simulink model "wt_multi"  (R2022b)
settings: Solver=FixedStepDiscrete  StartTime=0.0  StopTime=10.0  RelTol=1e-3
PreLoadFcn:
  | addpath('/nfs/ug/homes-1/z/zha13325/ece1718/a2_k/a2_hw/hdlimport/wt_multi');
libraries: simulink x2808, hdlsllib x1459
(part 10 of 22)

== system wt_multi/wt_multi/ca04/fa18 ==
  in1 : Inport  OutDataTypeStr=fixdt(0, 1, 0)  SampleTime=-1
  in2 : Inport  Port=2  OutDataTypeStr=fixdt(0, 1, 0)  SampleTime=-1
  Cin : Inport  Port=3  OutDataTypeStr=fixdt(0, 1, 0)  SampleTime=-1
  Bit_AND : simulink/Logic and Bit Operations/Bitwise Operator  logicop=AND  UseBitMask=off  NumInputPorts=2  BitMask=double(0)  BitMaskRealWorld=Real World Value
  Bit_AND_1 : simulink/Logic and Bit Operations/Bitwise Operator  logicop=AND  UseBitMask=off  NumInputPorts=2  BitMask=double(0)  BitMaskRealWorld=Real World Value
  Bit_OR : simulink/Logic and Bit Operations/Bitwise Operator  logicop=OR  UseBitMask=off  NumInputPorts=2  BitMask=double(0)  BitMaskRealWorld=Real World Value
  Bit_XOR : simulink/Logic and Bit Operations/Bitwise Operator  logicop=XOR  UseBitMask=off  NumInputPorts=2  BitMask=double(0)  BitMaskRealWorld=Real World Value
  Bit_XOR_1 : simulink/Logic and Bit Operations/Bitwise Operator  logicop=XOR  UseBitMask=off  NumInputPorts=2  BitMask=double(0)  BitMaskRealWorld=Real World Value
  Bit_XOR_2 : simulink/Logic and Bit Operations/Bitwise Operator  logicop=XOR  UseBitMask=off  NumInputPorts=2  BitMask=double(0)  BitMaskRealWorld=Real World Value
  S : Outport  OutDataTypeStr=fixdt(0, 1, 0)  SampleTime=-1
  C : Outport  Port=2  OutDataTypeStr=fixdt(0, 1, 0)  SampleTime=-1
  wires:
  in2/1 -> Bit_XOR_2/2, Bit_AND/2, Bit_XOR_1/2
  Cin/1 -> Bit_AND_1/1, Bit_XOR/2
  Bit_AND_1/1 -> Bit_OR/2
  in1/1 -> Bit_XOR_2/1, Bit_AND/1, Bit_XOR_1/1
  Bit_OR/1 -> C/1
  Bit_XOR_2/1 -> Bit_AND_1/2
  Bit_XOR/1 -> S/1
  Bit_AND/1 -> Bit_OR/1
  Bit_XOR_1/1 -> Bit_XOR/1

== system wt_multi/wt_multi/ca04/fa19 ==
  in1 : Inport  OutDataTypeStr=fixdt(0, 1, 0)  SampleTime=-1
  in2 : Inport  Port=2  OutDataTypeStr=fixdt(0, 1, 0)  SampleTime=-1
  Cin : Inport  Port=3  OutDataTypeStr=fixdt(0, 1, 0)  SampleTime=-1
  Bit_AND : simulink/Logic and Bit Operations/Bitwise Operator  logicop=AND  UseBitMask=off  NumInputPorts=2  BitMask=double(0)  BitMaskRealWorld=Real World Value
  Bit_AND_1 : simulink/Logic and Bit Operations/Bitwise Operator  logicop=AND  UseBitMask=off  NumInputPorts=2  BitMask=double(0)  BitMaskRealWorld=Real World Value
  Bit_OR : simulink/Logic and Bit Operations/Bitwise Operator  logicop=OR  UseBitMask=off  NumInputPorts=2  BitMask=double(0)  BitMaskRealWorld=Real World Value
  Bit_XOR : simulink/Logic and Bit Operations/Bitwise Operator  logicop=XOR  UseBitMask=off  NumInputPorts=2  BitMask=double(0)  BitMaskRealWorld=Real World Value
  Bit_XOR_1 : simulink/Logic and Bit Operations/Bitwise Operator  logicop=XOR  UseBitMask=off  NumInputPorts=2  BitMask=double(0)  BitMaskRealWorld=Real World Value
  Bit_XOR_2 : simulink/Logic and Bit Operations/Bitwise Operator  logicop=XOR  UseBitMask=off  NumInputPorts=2  BitMask=double(0)  BitMaskRealWorld=Real World Value
  S : Outport  OutDataTypeStr=fixdt(0, 1, 0)  SampleTime=-1
  C : Outport  Port=2  OutDataTypeStr=fixdt(0, 1, 0)  SampleTime=-1
  wires:
  in1/1 -> Bit_XOR_2/1, Bit_AND/1, Bit_XOR_1/1
  in2/1 -> Bit_XOR_2/2, Bit_AND/2, Bit_XOR_1/2
  Cin/1 -> Bit_AND_1/1, Bit_XOR/2
  Bit_AND_1/1 -> Bit_OR/2
  Bit_OR/1 -> C/1
  Bit_XOR_2/1 -> Bit_AND_1/2
  Bit_XOR/1 -> S/1
  Bit_AND/1 -> Bit_OR/1
  Bit_XOR_1/1 -> Bit_XOR/1

== system wt_multi/wt_multi/ca04/fa2 ==
  in1 : Inport  OutDataTypeStr=fixdt(0, 1, 0)  SampleTime=-1
  in2 : Inport  Port=2  OutDataTypeStr=fixdt(0, 1, 0)  SampleTime=-1
  Cin : Inport  Port=3  OutDataTypeStr=fixdt(0, 1, 0)  SampleTime=-1
  Bit_AND : simulink/Logic and Bit Operations/Bitwise Operator  logicop=AND  UseBitMask=off  NumInputPorts=2  BitMask=double(0)  BitMaskRealWorld=Real World Value
  Bit_AND_1 : simulink/Logic and Bit Operations/Bitwise Operator  logicop=AND  UseBitMask=off  NumInputPorts=2  BitMask=double(0)  BitMaskRealWorld=Real World Value
  Bit_OR : simulink/Logic and Bit Operations/Bitwise Operator  logicop=OR  UseBitMask=off  NumInputPorts=2  BitMask=double(0)  BitMaskRealWorld=Real World Value
  Bit_XOR : simulink/Logic and Bit Operations/Bitwise Operator  logicop=XOR  UseBitMask=off  NumInputPorts=2  BitMask=double(0)  BitMaskRealWorld=Real World Value
  Bit_XOR_1 : simulink/Logic and Bit Operations/Bitwise Operator  logicop=XOR  UseBitMask=off  NumInputPorts=2  BitMask=double(0)  BitMaskRealWorld=Real World Value
  Bit_XOR_2 : simulink/Logic and Bit Operations/Bitwise Operator  logicop=XOR  UseBitMask=off  NumInputPorts=2  BitMask=double(0)  BitMaskRealWorld=Real World Value
  S : Outport  OutDataTypeStr=fixdt(0, 1, 0)  SampleTime=-1
  C : Outport  Port=2  OutDataTypeStr=fixdt(0, 1, 0)  SampleTime=-1
  wires:
  in1/1 -> Bit_XOR_2/1, Bit_AND/1, Bit_XOR_1/1
  in2/1 -> Bit_XOR_2/2, Bit_AND/2, Bit_XOR_1/2
  Cin/1 -> Bit_AND_1/1, Bit_XOR/2
  Bit_AND_1/1 -> Bit_OR/2
  Bit_OR/1 -> C/1
  Bit_XOR_2/1 -> Bit_AND_1/2
  Bit_AND/1 -> Bit_OR/1
  Bit_XOR_1/1 -> Bit_XOR/1
  Bit_XOR/1 -> S/1

== system wt_multi/wt_multi/ca04/fa20 ==
  in1 : Inport  OutDataTypeStr=fixdt(0, 1, 0)  SampleTime=-1
  in2 : Inport  Port=2  OutDataTypeStr=fixdt(0, 1, 0)  SampleTime=-1
  Cin : Inport  Port=3  OutDataTypeStr=fixdt(0, 1, 0)  SampleTime=-1
  Bit_AND : simulink/Logic and Bit Operations/Bitwise Operator  logicop=AND  UseBitMask=off  NumInputPorts=2  BitMask=double(0)  BitMaskRealWorld=Real World Value
  Bit_AND_1 : simulink/Logic and Bit Operations/Bitwise Operator  logicop=AND  UseBitMask=off  NumInputPorts=2  BitMask=double(0)  BitMaskRealWorld=Real World Value
  Bit_OR : simulink/Logic and Bit Operations/Bitwise Operator  logicop=OR  UseBitMask=off  NumInputPorts=2  BitMask=double(0)  BitMaskRealWorld=Real World Value
  Bit_XOR : simulink/Logic and Bit Operations/Bitwise Operator  logicop=XOR  UseBitMask=off  NumInputPorts=2  BitMask=double(0)  BitMaskRealWorld=Real World Value
  Bit_XOR_1 : simulink/Logic and Bit Operations/Bitwise Operator  logicop=XOR  UseBitMask=off  NumInputPorts=2  BitMask=double(0)  BitMaskRealWorld=Real World Value
  Bit_XOR_2 : simulink/Logic and Bit Operations/Bitwise Operator  logicop=XOR  UseBitMask=off  NumInputPorts=2  BitMask=double(0)  BitMaskRealWorld=Real World Value
  S : Outport  OutDataTypeStr=fixdt(0, 1, 0)  SampleTime=-1
  C : Outport  Port=2  OutDataTypeStr=fixdt(0, 1, 0)  SampleTime=-1
  wires:
  in2/1 -> Bit_XOR_2/2, Bit_AND/2, Bit_XOR_1/2
  Bit_AND_1/1 -> Bit_OR/2
  Bit_OR/1 -> C/1
  Bit_XOR_1/1 -> Bit_XOR/1
  Bit_XOR_2/1 -> Bit_AND_1/2
  in1/1 -> Bit_XOR_2/1, Bit_AND/1, Bit_XOR_1/1
  Bit_AND/1 -> Bit_OR/1
  Cin/1 -> Bit_AND_1/1, Bit_XOR/2
  Bit_XOR/1 -> S/1

== system wt_multi/wt_multi/ca04/fa21 ==
  in1 : Inport  OutDataTypeStr=fixdt(0, 1, 0)  SampleTime=-1
  in2 : Inport  Port=2  OutDataTypeStr=fixdt(0, 1, 0)  SampleTime=-1
  Cin : Inport  Port=3  OutDataTypeStr=fixdt(0, 1, 0)  SampleTime=-1
  Bit_AND : simulink/Logic and Bit Operations/Bitwise Operator  logicop=AND  UseBitMask=off  NumInputPorts=2  BitMask=double(0)  BitMaskRealWorld=Real World Value
  Bit_AND_1 : simulink/Logic and Bit Operations/Bitwise Operator  logicop=AND  UseBitMask=off  NumInputPorts=2  BitMask=double(0)  BitMaskRealWorld=Real World Value
  Bit_OR : simulink/Logic and Bit Operations/Bitwise Operator  logicop=OR  UseBitMask=off  NumInputPorts=2  BitMask=double(0)  BitMaskRealWorld=Real World Value
  Bit_XOR : simulink/Logic and Bit Operations/Bitwise Operator  logicop=XOR  UseBitMask=off  NumInputPorts=2  BitMask=double(0)  BitMaskRealWorld=Real World Value
  Bit_XOR_1 : simulink/Logic and Bit Operations/Bitwise Operator  logicop=XOR  UseBitMask=off  NumInputPorts=2  BitMask=double(0)  BitMaskRealWorld=Real World Value
  Bit_XOR_2 : simulink/Logic and Bit Operations/Bitwise Operator  logicop=XOR  UseBitMask=off  NumInputPorts=2  BitMask=double(0)  BitMaskRealWorld=Real World Value
  S : Outport  OutDataTypeStr=fixdt(0, 1, 0)  SampleTime=-1
  C : Outport  Port=2  OutDataTypeStr=fixdt(0, 1, 0)  SampleTime=-1
  wires:
  in1/1 -> Bit_XOR_2/1, Bit_AND/1, Bit_XOR_1/1
  in2/1 -> Bit_XOR_2/2, Bit_AND/2, Bit_XOR_1/2
  Cin/1 -> Bit_AND_1/1, Bit_XOR/2
  Bit_AND_1/1 -> Bit_OR/2
  Bit_OR/1 -> C/1
  Bit_XOR_2/1 -> Bit_AND_1/2
  Bit_AND/1 -> Bit_OR/1
  Bit_XOR/1 -> S/1
  Bit_XOR_1/1 -> Bit_XOR/1

== system wt_multi/wt_multi/ca04/fa22 ==
  in1 : Inport  OutDataTypeStr=fixdt(0, 1, 0)  SampleTime=-1
  in2 : Inport  Port=2  OutDataTypeStr=fixdt(0, 1, 0)  SampleTime=-1
  Cin : Inport  Port=3  OutDataTypeStr=fixdt(0, 1, 0)  SampleTime=-1
  Bit_AND : simulink/Logic and Bit Operations/Bitwise Operator  logicop=AND  UseBitMask=off  NumInputPorts=2  BitMask=double(0)  BitMaskRealWorld=Real World Value
  Bit_AND_1 : simulink/Logic and Bit Operations/Bitwise Operator  logicop=AND  UseBitMask=off  NumInputPorts=2  BitMask=double(0)  BitMaskRealWorld=Real World Value
  Bit_OR : simulink/Logic and Bit Operations/Bitwise Operator  logicop=OR  UseBitMask=off  NumInputPorts=2  BitMask=double(0)  BitMaskRealWorld=Real World Value
  Bit_XOR : simulink/Logic and Bit Operations/Bitwise Operator  logicop=XOR  UseBitMask=off  NumInputPorts=2  BitMask=double(0)  BitMaskRealWorld=Real World Value
  Bit_XOR_1 : simulink/Logic and Bit Operations/Bitwise Operator  logicop=XOR  UseBitMask=off  NumInputPorts=2  BitMask=double(0)  BitMaskRealWorld=Real World Value
  Bit_XOR_2 : simulink/Logic and Bit Operations/Bitwise Operator  logicop=XOR  UseBitMask=off  NumInputPorts=2  BitMask=double(0)  BitMaskRealWorld=Real World Value
  S : Outport  OutDataTypeStr=fixdt(0, 1, 0)  SampleTime=-1
  C : Outport  Port=2  OutDataTypeStr=fixdt(0, 1, 0)  SampleTime=-1
  wires:
  in1/1 -> Bit_XOR_2/1, Bit_AND/1, Bit_XOR_1/1
  in2/1 -> Bit_XOR_2/2, Bit_AND/2, Bit_XOR_1/2
  Bit_AND_1/1 -> Bit_OR/2
  Bit_OR/1 -> C/1
  Cin/1 -> Bit_AND_1/1, Bit_XOR/2
  Bit_AND/1 -> Bit_OR/1
  Bit_XOR_2/1 -> Bit_AND_1/2
  Bit_XOR/1 -> S/1
  Bit_XOR_1/1 -> Bit_XOR/1

== system wt_multi/wt_multi/ca04/fa23 ==
  in1 : Inport  OutDataTypeStr=fixdt(0, 1, 0)  SampleTime=-1
  in2 : Inport  Port=2  OutDataTypeStr=fixdt(0, 1, 0)  SampleTime=-1
  Cin : Inport  Port=3  OutDataTypeStr=fixdt(0, 1, 0)  SampleTime=-1
  Bit_AND : simulink/Logic and Bit Operations/Bitwise Operator  logicop=AND  UseBitMask=off  NumInputPorts=2  BitMask=double(0)  BitMaskRealWorld=Real World Value
  Bit_AND_1 : simulink/Logic and Bit Operations/Bitwise Operator  logicop=AND  UseBitMask=off  NumInputPorts=2  BitMask=double(0)  BitMaskRealWorld=Real World Value
  Bit_OR : simulink/Logic and Bit Operations/Bitwise Operator  logicop=OR  UseBitMask=off  NumInputPorts=2  BitMask=double(0)  BitMaskRealWorld=Real World Value
  Bit_XOR : simulink/Logic and Bit Operations/Bitwise Operator  logicop=XOR  UseBitMask=off  NumInputPorts=2  BitMask=double(0)  BitMaskRealWorld=Real World Value
  Bit_XOR_1 : simulink/Logic and Bit Operations/Bitwise Operator  logicop=XOR  UseBitMask=off  NumInputPorts=2  BitMask=double(0)  BitMaskRealWorld=Real World Value
  Bit_XOR_2 : simulink/Logic and Bit Operations/Bitwise Operator  logicop=XOR  UseBitMask=off  NumInputPorts=2  BitMask=double(0)  BitMaskRealWorld=Real World Value
  S : Outport  OutDataTypeStr=fixdt(0, 1, 0)  SampleTime=-1
  C : Outport  Port=2  OutDataTypeStr=fixdt(0, 1, 0)  SampleTime=-1
  wires:
  in1/1 -> Bit_XOR_2/1, Bit_AND/1, Bit_XOR_1/1
  in2/1 -> Bit_XOR_2/2, Bit_AND/2, Bit_XOR_1/2
  Bit_AND_1/1 -> Bit_OR/2
  Bit_OR/1 -> C/1
  Bit_XOR_2/1 -> Bit_AND_1/2
  Bit_XOR_1/1 -> Bit_XOR/1
  Cin/1 -> Bit_AND_1/1, Bit_XOR/2
  Bit_AND/1 -> Bit_OR/1
  Bit_XOR/1 -> S/1

== system wt_multi/wt_multi/ca04/fa24 ==
  in1 : Inport  OutDataTypeStr=fixdt(0, 1, 0)  SampleTime=-1
  in2 : Inport  Port=2  OutDataTypeStr=fixdt(0, 1, 0)  SampleTime=-1
  Cin : Inport  Port=3  OutDataTypeStr=fixdt(0, 1, 0)  SampleTime=-1
  Bit_AND : simulink/Logic and Bit Operations/Bitwise Operator  logicop=AND  UseBitMask=off  NumInputPorts=2  BitMask=double(0)  BitMaskRealWorld=Real World Value
  Bit_AND_1 : simulink/Logic and Bit Operations/Bitwise Operator  logicop=AND  UseBitMask=off  NumInputPorts=2  BitMask=double(0)  BitMaskRealWorld=Real World Value
  Bit_OR : simulink/Logic and Bit Operations/Bitwise Operator  logicop=OR  UseBitMask=off  NumInputPorts=2  BitMask=double(0)  BitMaskRealWorld=Real World Value
  Bit_XOR : simulink/Logic and Bit Operations/Bitwise Operator  logicop=XOR  UseBitMask=off  NumInputPorts=2  BitMask=double(0)  BitMaskRealWorld=Real World Value
  Bit_XOR_1 : simulink/Logic and Bit Operations/Bitwise Operator  logicop=XOR  UseBitMask=off  NumInputPorts=2  BitMask=double(0)  BitMaskRealWorld=Real World Value
  Bit_XOR_2 : simulink/Logic and Bit Operations/Bitwise Operator  logicop=XOR  UseBitMask=off  NumInputPorts=2  BitMask=double(0)  BitMaskRealWorld=Real World Value
  S : Outport  OutDataTypeStr=fixdt(0, 1, 0)  SampleTime=-1
  C : Outport  Port=2  OutDataTypeStr=fixdt(0, 1, 0)  SampleTime=-1
  wires:
  in1/1 -> Bit_XOR_2/1, Bit_AND/1, Bit_XOR_1/1
  Cin/1 -> Bit_AND_1/1, Bit_XOR/2
  Bit_AND_1/1 -> Bit_OR/2
  Bit_XOR_1/1 -> Bit_XOR/1
  in2/1 -> Bit_XOR_2/2, Bit_AND/2, Bit_XOR_1/2
  Bit_OR/1 -> C/1
  Bit_XOR/1 -> S/1
  Bit_XOR_2/1 -> Bit_AND_1/2
  Bit_AND/1 -> Bit_OR/1

== system wt_multi/wt_multi/ca04/fa25 ==
  in1 : Inport  OutDataTypeStr=fixdt(0, 1, 0)  SampleTime=-1
  in2 : Inport  Port=2  OutDataTypeStr=fixdt(0, 1, 0)  SampleTime=-1
  Cin : Inport  Port=3  OutDataTypeStr=fixdt(0, 1, 0)  SampleTime=-1
  Bit_AND : simulink/Logic and Bit Operations/Bitwise Operator  logicop=AND  UseBitMask=off  NumInputPorts=2  BitMask=double(0)  BitMaskRealWorld=Real World Value
  Bit_AND_1 : simulink/Logic and Bit Operations/Bitwise Operator  logicop=AND  UseBitMask=off  NumInputPorts=2  BitMask=double(0)  BitMaskRealWorld=Real World Value
  Bit_OR : simulink/Logic and Bit Operations/Bitwise Operator  logicop=OR  UseBitMask=off  NumInputPorts=2  BitMask=double(0)  BitMaskRealWorld=Real World Value
  Bit_XOR : simulink/Logic and Bit Operations/Bitwise Operator  logicop=XOR  UseBitMask=off  NumInputPorts=2  BitMask=double(0)  BitMaskRealWorld=Real World Value
  Bit_XOR_1 : simulink/Logic and Bit Operations/Bitwise Operator  logicop=XOR  UseBitMask=off  NumInputPorts=2  BitMask=double(0)  BitMaskRealWorld=Real World Value
  Bit_XOR_2 : simulink/Logic and Bit Operations/Bitwise Operator  logicop=XOR  UseBitMask=off  NumInputPorts=2  BitMask=double(0)  BitMaskRealWorld=Real World Value
  S : Outport  OutDataTypeStr=fixdt(0, 1, 0)  SampleTime=-1
  C : Outport  Port=2  OutDataTypeStr=fixdt(0, 1, 0)  SampleTime=-1
  wires:
  in1/1 -> Bit_XOR_2/1, Bit_AND/1, Bit_XOR_1/1
  in2/1 -> Bit_XOR_2/2, Bit_AND/2, Bit_XOR_1/2
  Cin/1 -> Bit_AND_1/1, Bit_XOR/2
  Bit_AND_1/1 -> Bit_OR/2
  Bit_AND/1 -> Bit_OR/1
  Bit_OR/1 -> C/1
  Bit_XOR_1/1 -> Bit_XOR/1
  Bit_XOR_2/1 -> Bit_AND_1/2
  Bit_XOR/1 -> S/1

== system wt_multi/wt_multi/ca04/fa26 ==
  in1 : Inport  OutDataTypeStr=fixdt(0, 1, 0)  SampleTime=-1
  in2 : Inport  Port=2  OutDataTypeStr=fixdt(0, 1, 0)  SampleTime=-1
  Cin : Inport  Port=3  OutDataTypeStr=fixdt(0, 1, 0)  SampleTime=-1
  Bit_AND : simulink/Logic and Bit Operations/Bitwise Operator  logicop=AND  UseBitMask=off  NumInputPorts=2  BitMask=double(0)  BitMaskRealWorld=Real World Value
  Bit_AND_1 : simulink/Logic and Bit Operations/Bitwise Operator  logicop=AND  UseBitMask=off  NumInputPorts=2  BitMask=double(0)  BitMaskRealWorld=Real World Value
  Bit_OR : simulink/Logic and Bit Operations/Bitwise Operator  logicop=OR  UseBitMask=off  NumInputPorts=2  BitMask=double(0)  BitMaskRealWorld=Real World Value
  Bit_XOR : simulink/Logic and Bit Operations/Bitwise Operator  logicop=XOR  UseBitMask=off  NumInputPorts=2  BitMask=double(0)  BitMaskRealWorld=Real World Value
  Bit_XOR_1 : simulink/Logic and Bit Operations/Bitwise Operator  logicop=XOR  UseBitMask=off  NumInputPorts=2  BitMask=double(0)  BitMaskRealWorld=Real World Value
  Bit_XOR_2 : simulink/Logic and Bit Operations/Bitwise Operator  logicop=XOR  UseBitMask=off  NumInputPorts=2  BitMask=double(0)  BitMaskRealWorld=Real World Value
  S : Outport  OutDataTypeStr=fixdt(0, 1, 0)  SampleTime=-1
  C : Outport  Port=2  OutDataTypeStr=fixdt(0, 1, 0)  SampleTime=-1
  wires:
  in1/1 -> Bit_XOR_2/1, Bit_AND/1, Bit_XOR_1/1
  in2/1 -> Bit_XOR_2/2, Bit_AND/2, Bit_XOR_1/2
  Cin/1 -> Bit_AND_1/1, Bit_XOR/2
  Bit_OR/1 -> C/1
  Bit_AND/1 -> Bit_OR/1
  Bit_XOR/1 -> S/1
  Bit_AND_1/1 -> Bit_OR/2
  Bit_XOR_2/1 -> Bit_AND_1/2
  Bit_XOR_1/1 -> Bit_XOR/1

== system wt_multi/wt_multi/ca04/fa27 ==
  in1 : Inport  OutDataTypeStr=fixdt(0, 1, 0)  SampleTime=-1
  in2 : Inport  Port=2  OutDataTypeStr=fixdt(0, 1, 0)  SampleTime=-1
  Cin : Inport  Port=3  OutDataTypeStr=fixdt(0, 1, 0)  SampleTime=-1
  Bit_AND : simulink/Logic and Bit Operations/Bitwise Operator  logicop=AND  UseBitMask=off  NumInputPorts=2  BitMask=double(0)  BitMaskRealWorld=Real World Value
  Bit_AND_1 : simulink/Logic and Bit Operations/Bitwise Operator  logicop=AND  UseBitMask=off  NumInputPorts=2  BitMask=double(0)  BitMaskRealWorld=Real World Value
  Bit_OR : simulink/Logic and Bit Operations/Bitwise Operator  logicop=OR  UseBitMask=off  NumInputPorts=2  BitMask=double(0)  BitMaskRealWorld=Real World Value
  Bit_XOR : simulink/Logic and Bit Operations/Bitwise Operator  logicop=XOR  UseBitMask=off  NumInputPorts=2  BitMask=double(0)  BitMaskRealWorld=Real World Value
  Bit_XOR_1 : simulink/Logic and Bit Operations/Bitwise Operator  logicop=XOR  UseBitMask=off  NumInputPorts=2  BitMask=double(0)  BitMaskRealWorld=Real World Value
  Bit_XOR_2 : simulink/Logic and Bit Operations/Bitwise Operator  logicop=XOR  UseBitMask=off  NumInputPorts=2  BitMask=double(0)  BitMaskRealWorld=Real World Value
  S : Outport  OutDataTypeStr=fixdt(0, 1, 0)  SampleTime=-1
  C : Outport  Port=2  OutDataTypeStr=fixdt(0, 1, 0)  SampleTime=-1
  wires:
  in1/1 -> Bit_XOR_2/1, Bit_AND/1, Bit_XOR_1/1
  in2/1 -> Bit_XOR_2/2, Bit_AND/2, Bit_XOR_1/2
  Cin/1 -> Bit_AND_1/1, Bit_XOR/2
  Bit_AND_1/1 -> Bit_OR/2
  Bit_XOR_2/1 -> Bit_AND_1/2
  Bit_OR/1 -> C/1
  Bit_XOR_1/1 -> Bit_XOR/1
  Bit_AND/1 -> Bit_OR/1
  Bit_XOR/1 -> S/1

== system wt_multi/wt_multi/ca04/fa28 ==
  in1 : Inport  OutDataTypeStr=fixdt(0, 1, 0)  SampleTime=-1
  in2 : Inport  Port=2  OutDataTypeStr=fixdt(0, 1, 0)  SampleTime=-1
  Cin : Inport  Port=3  OutDataTypeStr=fixdt(0, 1, 0)  SampleTime=-1
  Bit_AND : simulink/Logic and Bit Operations/Bitwise Operator  logicop=AND  UseBitMask=off  NumInputPorts=2  BitMask=double(0)  BitMaskRealWorld=Real World Value
  Bit_AND_1 : simulink/Logic and Bit Operations/Bitwise Operator  logicop=AND  UseBitMask=off  NumInputPorts=2  BitMask=double(0)  BitMaskRealWorld=Real World Value
  Bit_OR : simulink/Logic and Bit Operations/Bitwise Operator  logicop=OR  UseBitMask=off  NumInputPorts=2  BitMask=double(0)  BitMaskRealWorld=Real World Value
  Bit_XOR : simulink/Logic and Bit Operations/Bitwise Operator  logicop=XOR  UseBitMask=off  NumInputPorts=2  BitMask=double(0)  BitMaskRealWorld=Real World Value
  Bit_XOR_1 : simulink/Logic and Bit Operations/Bitwise Operator  logicop=XOR  UseBitMask=off  NumInputPorts=2  BitMask=double(0)  BitMaskRealWorld=Real World Value
  Bit_XOR_2 : simulink/Logic and Bit Operations/Bitwise Operator  logicop=XOR  UseBitMask=off  NumInputPorts=2  BitMask=double(0)  BitMaskRealWorld=Real World Value
  S : Outport  OutDataTypeStr=fixdt(0, 1, 0)  SampleTime=-1
  C : Outport  Port=2  OutDataTypeStr=fixdt(0, 1, 0)  SampleTime=-1
  wires:
  Cin/1 -> Bit_AND_1/1, Bit_XOR/2
  Bit_AND/1 -> Bit_OR/1
  Bit_OR/1 -> C/1
  in1/1 -> Bit_XOR_2/1, Bit_AND/1, Bit_XOR_1/1
  Bit_AND_1/1 -> Bit_OR/2
  Bit_XOR_2/1 -> Bit_AND_1/2
  Bit_XOR/1 -> S/1
  in2/1 -> Bit_XOR_2/2, Bit_AND/2, Bit_XOR_1/2
  Bit_XOR_1/1 -> Bit_XOR/1

== system wt_multi/wt_multi/ca04/fa29 ==
  in1 : Inport  OutDataTypeStr=fixdt(0, 1, 0)  SampleTime=-1
  in2 : Inport  Port=2  OutDataTypeStr=fixdt(0, 1, 0)  SampleTime=-1
  Cin : Inport  Port=3  OutDataTypeStr=fixdt(0, 1, 0)  SampleTime=-1
  Bit_AND : simulink/Logic and Bit Operations/Bitwise Operator  logicop=AND  UseBitMask=off  NumInputPorts=2  BitMask=double(0)  BitMaskRealWorld=Real World Value
  Bit_AND_1 : simulink/Logic and Bit Operations/Bitwise Operator  logicop=AND  UseBitMask=off  NumInputPorts=2  BitMask=double(0)  BitMaskRealWorld=Real World Value
  Bit_OR : simulink/Logic and Bit Operations/Bitwise Operator  logicop=OR  UseBitMask=off  NumInputPorts=2  BitMask=double(0)  BitMaskRealWorld=Real World Value
  Bit_XOR : simulink/Logic and Bit Operations/Bitwise Operator  logicop=XOR  UseBitMask=off  NumInputPorts=2  BitMask=double(0)  BitMaskRealWorld=Real World Value
  Bit_XOR_1 : simulink/Logic and Bit Operations/Bitwise Operator  logicop=XOR  UseBitMask=off  NumInputPorts=2  BitMask=double(0)  BitMaskRealWorld=Real World Value
  Bit_XOR_2 : simulink/Logic and Bit Operations/Bitwise Operator  logicop=XOR  UseBitMask=off  NumInputPorts=2  BitMask=double(0)  BitMaskRealWorld=Real World Value
  S : Outport  OutDataTypeStr=fixdt(0, 1, 0)  SampleTime=-1
  C : Outport  Port=2  OutDataTypeStr=fixdt(0, 1, 0)  SampleTime=-1
  wires:
  in2/1 -> Bit_XOR_2/2, Bit_AND/2, Bit_XOR_1/2
  Cin/1 -> Bit_AND_1/1, Bit_XOR/2
  Bit_AND/1 -> Bit_OR/1
  Bit_AND_1/1 -> Bit_OR/2
  Bit_OR/1 -> C/1
  Bit_XOR/1 -> S/1
  in1/1 -> Bit_XOR_2/1, Bit_AND/1, Bit_XOR_1/1
  Bit_XOR_2/1 -> Bit_AND_1/2
  Bit_XOR_1/1 -> Bit_XOR/1

== system wt_multi/wt_multi/ca04/fa3 ==
  in1 : Inport  OutDataTypeStr=fixdt(0, 1, 0)  SampleTime=-1
  in2 : Inport  Port=2  OutDataTypeStr=fixdt(0, 1, 0)  SampleTime=-1
  Cin : Inport  Port=3  OutDataTypeStr=fixdt(0, 1, 0)  SampleTime=-1
  Bit_AND : simulink/Logic and Bit Operations/Bitwise Operator  logicop=AND  UseBitMask=off  NumInputPorts=2  BitMask=double(0)  BitMaskRealWorld=Real World Value
  Bit_AND_1 : simulink/Logic and Bit Operations/Bitwise Operator  logicop=AND  UseBitMask=off  NumInputPorts=2  BitMask=double(0)  BitMaskRealWorld=Real World Value
  Bit_OR : simulink/Logic and Bit Operations/Bitwise Operator  logicop=OR  UseBitMask=off  NumInputPorts=2  BitMask=double(0)  BitMaskRealWorld=Real World Value
  Bit_XOR : simulink/Logic and Bit Operations/Bitwise Operator  logicop=XOR  UseBitMask=off  NumInputPorts=2  BitMask=double(0)  BitMaskRealWorld=Real World Value
  Bit_XOR_1 : simulink/Logic and Bit Operations/Bitwise Operator  logicop=XOR  UseBitMask=off  NumInputPorts=2  BitMask=double(0)  BitMaskRealWorld=Real World Value
  Bit_XOR_2 : simulink/Logic and Bit Operations/Bitwise Operator  logicop=XOR  UseBitMask=off  NumInputPorts=2  BitMask=double(0)  BitMaskRealWorld=Real World Value
  S : Outport  OutDataTypeStr=fixdt(0, 1, 0)  SampleTime=-1
  C : Outport  Port=2  OutDataTypeStr=fixdt(0, 1, 0)  SampleTime=-1
  wires:
  in1/1 -> Bit_XOR_2/1, Bit_AND/1, Bit_XOR_1/1
  Cin/1 -> Bit_AND_1/1, Bit_XOR/2
  Bit_AND_1/1 -> Bit_OR/2
  Bit_XOR_2/1 -> Bit_AND_1/2
  Bit_OR/1 -> C/1
  in2/1 -> Bit_XOR_2/2, Bit_AND/2, Bit_XOR_1/2
  Bit_XOR/1 -> S/1
  Bit_XOR_1/1 -> Bit_XOR/1
  Bit_AND/1 -> Bit_OR/1

== system wt_multi/wt_multi/ca04/fa30 ==
  in1 : Inport  OutDataTypeStr=fixdt(0, 1, 0)  SampleTime=-1
  in2 : Inport  Port=2  OutDataTypeStr=fixdt(0, 1, 0)  SampleTime=-1
  Cin : Inport  Port=3  OutDataTypeStr=fixdt(0, 1, 0)  SampleTime=-1
  Bit_AND : simulink/Logic and Bit Operations/Bitwise Operator  logicop=AND  UseBitMask=off  NumInputPorts=2  BitMask=double(0)  BitMaskRealWorld=Real World Value
  Bit_AND_1 : simulink/Logic and Bit Operations/Bitwise Operator  logicop=AND  UseBitMask=off  NumInputPorts=2  BitMask=double(0)  BitMaskRealWorld=Real World Value
  Bit_OR : simulink/Logic and Bit Operations/Bitwise Operator  logicop=OR  UseBitMask=off  NumInputPorts=2  BitMask=double(0)  BitMaskRealWorld=Real World Value
  Bit_XOR : simulink/Logic and Bit Operations/Bitwise Operator  logicop=XOR  UseBitMask=off  NumInputPorts=2  BitMask=double(0)  BitMaskRealWorld=Real World Value
  Bit_XOR_1 : simulink/Logic and Bit Operations/Bitwise Operator  logicop=XOR  UseBitMask=off  NumInputPorts=2  BitMask=double(0)  BitMaskRealWorld=Real World Value
  Bit_XOR_2 : simulink/Logic and Bit Operations/Bitwise Operator  logicop=XOR  UseBitMask=off  NumInputPorts=2  BitMask=double(0)  BitMaskRealWorld=Real World Value
  S : Outport  OutDataTypeStr=fixdt(0, 1, 0)  SampleTime=-1
  C : Outport  Port=2  OutDataTypeStr=fixdt(0, 1, 0)  SampleTime=-1
  wires:
  in1/1 -> Bit_XOR_2/1, Bit_AND/1, Bit_XOR_1/1
  in2/1 -> Bit_XOR_2/2, Bit_AND/2, Bit_XOR_1/2
  Cin/1 -> Bit_AND_1/1, Bit_XOR/2
  Bit_AND_1/1 -> Bit_OR/2
  Bit_OR/1 -> C/1
  Bit_XOR_1/1 -> Bit_XOR/1
  Bit_XOR_2/1 -> Bit_AND_1/2
  Bit_AND/1 -> Bit_OR/1
  Bit_XOR/1 -> S/1

== system wt_multi/wt_multi/ca04/fa4 ==
  in1 : Inport  OutDataTypeStr=fixdt(0, 1, 0)  SampleTime=-1
  in2 : Inport  Port=2  OutDataTypeStr=fixdt(0, 1, 0)  SampleTime=-1
  Cin : Inport  Port=3  OutDataTypeStr=fixdt(0, 1, 0)  SampleTime=-1
  Bit_AND : simulink/Logic and Bit Operations/Bitwise Operator  logicop=AND  UseBitMask=off  NumInputPorts=2  BitMask=double(0)  BitMaskRealWorld=Real World Value
  Bit_AND_1 : simulink/Logic and Bit Operations/Bitwise Operator  logicop=AND  UseBitMask=off  NumInputPorts=2  BitMask=double(0)  BitMaskRealWorld=Real World Value
  Bit_OR : simulink/Logic and Bit Operations/Bitwise Operator  logicop=OR  UseBitMask=off  NumInputPorts=2  BitMask=double(0)  BitMaskRealWorld=Real World Value
  Bit_XOR : simulink/Logic and Bit Operations/Bitwise Operator  logicop=XOR  UseBitMask=off  NumInputPorts=2  BitMask=double(0)  BitMaskRealWorld=Real World Value
  Bit_XOR_1 : simulink/Logic and Bit Operations/Bitwise Operator  logicop=XOR  UseBitMask=off  NumInputPorts=2  BitMask=double(0)  BitMaskRealWorld=Real World Value
  Bit_XOR_2 : simulink/Logic and Bit Operations/Bitwise Operator  logicop=XOR  UseBitMask=off  NumInputPorts=2  BitMask=double(0)  BitMaskRealWorld=Real World Value
  S : Outport  OutDataTypeStr=fixdt(0, 1, 0)  SampleTime=-1
  C : Outport  Port=2  OutDataTypeStr=fixdt(0, 1, 0)  SampleTime=-1
  wires:
  Cin/1 -> Bit_AND_1/1, Bit_XOR/2
  Bit_AND_1/1 -> Bit_OR/2
  Bit_OR/1 -> C/1
  Bit_XOR_2/1 -> Bit_AND_1/2
  Bit_AND/1 -> Bit_OR/1
  in1/1 -> Bit_XOR_2/1, Bit_AND/1, Bit_XOR_1/1
  in2/1 -> Bit_XOR_2/2, Bit_AND/2, Bit_XOR_1/2
  Bit_XOR/1 -> S/1
  Bit_XOR_1/1 -> Bit_XOR/1

== system wt_multi/wt_multi/ca04/fa5 ==
  in1 : Inport  OutDataTypeStr=fixdt(0, 1, 0)  SampleTime=-1
  in2 : Inport  Port=2  OutDataTypeStr=fixdt(0, 1, 0)  SampleTime=-1
  Cin : Inport  Port=3  OutDataTypeStr=fixdt(0, 1, 0)  SampleTime=-1
  Bit_AND : simulink/Logic and Bit Operations/Bitwise Operator  logicop=AND  UseBitMask=off  NumInputPorts=2  BitMask=double(0)  BitMaskRealWorld=Real World Value
  Bit_AND_1 : simulink/Logic and Bit Operations/Bitwise Operator  logicop=AND  UseBitMask=off  NumInputPorts=2  BitMask=double(0)  BitMaskRealWorld=Real World Value
  Bit_OR : simulink/Logic and Bit Operations/Bitwise Operator  logicop=OR  UseBitMask=off  NumInputPorts=2  BitMask=double(0)  BitMaskRealWorld=Real World Value
  Bit_XOR : simulink/Logic and Bit Operations/Bitwise Operator  logicop=XOR  UseBitMask=off  NumInputPorts=2  BitMask=double(0)  BitMaskRealWorld=Real World Value
  Bit_XOR_1 : simulink/Logic and Bit Operations/Bitwise Operator  logicop=XOR  UseBitMask=off  NumInputPorts=2  BitMask=double(0)  BitMaskRealWorld=Real World Value
  Bit_XOR_2 : simulink/Logic and Bit Operations/Bitwise Operator  logicop=XOR  UseBitMask=off  NumInputPorts=2  BitMask=double(0)  BitMaskRealWorld=Real World Value
  S : Outport  OutDataTypeStr=fixdt(0, 1, 0)  SampleTime=-1
  C : Outport  Port=2  OutDataTypeStr=fixdt(0, 1, 0)  SampleTime=-1
  wires:
  in2/1 -> Bit_XOR_2/2, Bit_AND/2, Bit_XOR_1/2
  Cin/1 -> Bit_AND_1/1, Bit_XOR/2
  Bit_AND_1/1 -> Bit_OR/2
  Bit_OR/1 -> C/1
  Bit_XOR_2/1 -> Bit_AND_1/2
  in1/1 -> Bit_XOR_2/1, Bit_AND/1, Bit_XOR_1/1
  Bit_AND/1 -> Bit_OR/1
  Bit_XOR_1/1 -> Bit_XOR/1
  Bit_XOR/1 -> S/1

== system wt_multi/wt_multi/ca04/fa6 ==
  in1 : Inport  OutDataTypeStr=fixdt(0, 1, 0)  SampleTime=-1
  in2 : Inport  Port=2  OutDataTypeStr=fixdt(0, 1, 0)  SampleTime=-1
  Cin : Inport  Port=3  OutDataTypeStr=fixdt(0, 1, 0)  SampleTime=-1
  Bit_AND : simulink/Logic and Bit Operations/Bitwise Operator  logicop=AND  UseBitMask=off  NumInputPorts=2  BitMask=double(0)  BitMaskRealWorld=Real World Value
  Bit_AND_1 : simulink/Logic and Bit Operations/Bitwise Operator  logicop=AND  UseBitMask=off  NumInputPorts=2  BitMask=double(0)  BitMaskRealWorld=Real World Value
  Bit_OR : simulink/Logic and Bit Operations/Bitwise Operator  logicop=OR  UseBitMask=off  NumInputPorts=2  BitMask=double(0)  BitMaskRealWorld=Real World Value
  Bit_XOR : simulink/Logic and Bit Operations/Bitwise Operator  logicop=XOR  UseBitMask=off  NumInputPorts=2  BitMask=double(0)  BitMaskRealWorld=Real World Value
  Bit_XOR_1 : simulink/Logic and Bit Operations/Bitwise Operator  logicop=XOR  UseBitMask=off  NumInputPorts=2  BitMask=double(0)  BitMaskRealWorld=Real World Value
  Bit_XOR_2 : simulink/Logic and Bit Operations/Bitwise Operator  logicop=XOR  UseBitMask=off  NumInputPorts=2  BitMask=double(0)  BitMaskRealWorld=Real World Value
  S : Outport  OutDataTypeStr=fixdt(0, 1, 0)  SampleTime=-1
  C : Outport  Port=2  OutDataTypeStr=fixdt(0, 1, 0)  SampleTime=-1
  wires:
  in1/1 -> Bit_XOR_2/1, Bit_AND/1, Bit_XOR_1/1
  Bit_AND_1/1 -> Bit_OR/2
  in2/1 -> Bit_XOR_2/2, Bit_AND/2, Bit_XOR_1/2
  Cin/1 -> Bit_AND_1/1, Bit_XOR/2
  Bit_OR/1 -> C/1
  Bit_XOR_2/1 -> Bit_AND_1/2
  Bit_AND/1 -> Bit_OR/1
  Bit_XOR/1 -> S/1
  Bit_XOR_1/1 -> Bit_XOR/1

== system wt_multi/wt_multi/ca04/fa7 ==
  in1 : Inport  OutDataTypeStr=fixdt(0, 1, 0)  SampleTime=-1
  in2 : Inport  Port=2  OutDataTypeStr=fixdt(0, 1, 0)  SampleTime=-1
  Cin : Inport  Port=3  OutDataTypeStr=fixdt(0, 1, 0)  SampleTime=-1
  Bit_AND : simulink/Logic and Bit Operations/Bitwise Operator  logicop=AND  UseBitMask=off  NumInputPorts=2  BitMask=double(0)  BitMaskRealWorld=Real World Value
  Bit_AND_1 : simulink/Logic and Bit Operations/Bitwise Operator  logicop=AND  UseBitMask=off  NumInputPorts=2  BitMask=double(0)  BitMaskRealWorld=Real World Value
  Bit_OR : simulink/Logic and Bit Operations/Bitwise Operator  logicop=OR  UseBitMask=off  NumInputPorts=2  BitMask=double(0)  BitMaskRealWorld=Real World Value
  Bit_XOR : simulink/Logic and Bit Operations/Bitwise Operator  logicop=XOR  UseBitMask=off  NumInputPorts=2  BitMask=double(0)  BitMaskRealWorld=Real World Value
  Bit_XOR_1 : simulink/Logic and Bit Operations/Bitwise Operator  logicop=XOR  UseBitMask=off  NumInputPorts=2  BitMask=double(0)  BitMaskRealWorld=Real World Value
  Bit_XOR_2 : simulink/Logic and Bit Operations/Bitwise Operator  logicop=XOR  UseBitMask=off  NumInputPorts=2  BitMask=double(0)  BitMaskRealWorld=Real World Value
  S : Outport  OutDataTypeStr=fixdt(0, 1, 0)  SampleTime=-1
  C : Outport  Port=2  OutDataTypeStr=fixdt(0, 1, 0)  SampleTime=-1
  wires:
  in1/1 -> Bit_XOR_2/1, Bit_AND/1, Bit_XOR_1/1
  in2/1 -> Bit_XOR_2/2, Bit_AND/2, Bit_XOR_1/2
  Cin/1 -> Bit_AND_1/1, Bit_XOR/2
  Bit_AND_1/1 -> Bit_OR/2
  Bit_OR/1 -> C/1
  Bit_XOR_2/1 -> Bit_AND_1/2
  Bit_XOR_1/1 -> Bit_XOR/1
  Bit_AND/1 -> Bit_OR/1
  Bit_XOR/1 -> S/1

== system wt_multi/wt_multi/ca04/fa8 ==
  in1 : Inport  OutDataTypeStr=fixdt(0, 1, 0)  SampleTime=-1
  in2 : Inport  Port=2  OutDataTypeStr=fixdt(0, 1, 0)  SampleTime=-1
  Cin : Inport  Port=3  OutDataTypeStr=fixdt(0, 1, 0)  SampleTime=-1
  Bit_AND : simulink/Logic and Bit Operations/Bitwise Operator  logicop=AND  UseBitMask=off  NumInputPorts=2  BitMask=double(0)  BitMaskRealWorld=Real World Value
  Bit_AND_1 : simulink/Logic and Bit Operations/Bitwise Operator  logicop=AND  UseBitMask=off  NumInputPorts=2  BitMask=double(0)  BitMaskRealWorld=Real World Value
  Bit_OR : simulink/Logic and Bit Operations/Bitwise Operator  logicop=OR  UseBitMask=off  NumInputPorts=2  BitMask=double(0)  BitMaskRealWorld=Real World Value
  Bit_XOR : simulink/Logic and Bit Operations/Bitwise Operator  logicop=XOR  UseBitMask=off  NumInputPorts=2  BitMask=double(0)  BitMaskRealWorld=Real World Value
  Bit_XOR_1 : simulink/Logic and Bit Operations/Bitwise Operator  logicop=XOR  UseBitMask=off  NumInputPorts=2  BitMask=double(0)  BitMaskRealWorld=Real World Value
  Bit_XOR_2 : simulink/Logic and Bit Operations/Bitwise Operator  logicop=XOR  UseBitMask=off  NumInputPorts=2  BitMask=double(0)  BitMaskRealWorld=Real World Value
  S : Outport  OutDataTypeStr=fixdt(0, 1, 0)  SampleTime=-1
  C : Outport  Port=2  OutDataTypeStr=fixdt(0, 1, 0)  SampleTime=-1
  wires:
  in1/1 -> Bit_XOR_2/1, Bit_AND/1, Bit_XOR_1/1
  Cin/1 -> Bit_AND_1/1, Bit_XOR/2
  Bit_AND_1/1 -> Bit_OR/2
  in2/1 -> Bit_XOR_2/2, Bit_AND/2, Bit_XOR_1/2
  Bit_AND/1 -> Bit_OR/1
  Bit_OR/1 -> C/1
  Bit_XOR_2/1 -> Bit_AND_1/2
  Bit_XOR/1 -> S/1
  Bit_XOR_1/1 -> Bit_XOR/1

== system wt_multi/wt_multi/ca04/fa9 ==
  in1 : Inport  OutDataTypeStr=fixdt(0, 1, 0)  SampleTime=-1
  in2 : Inport  Port=2  OutDataTypeStr=fixdt(0, 1, 0)  SampleTime=-1
  Cin : Inport  Port=3  OutDataTypeStr=fixdt(0, 1, 0)  SampleTime=-1
  Bit_AND : simulink/Logic and Bit Operations/Bitwise Operator  logicop=AND  UseBitMask=off  NumInputPorts=2  BitMask=double(0)  BitMaskRealWorld=Real World Value
  Bit_AND_1 : simulink/Logic and Bit Operations/Bitwise Operator  logicop=AND  UseBitMask=off  NumInputPorts=2  BitMask=double(0)  BitMaskRealWorld=Real World Value
  Bit_OR : simulink/Logic and Bit Operations/Bitwise Operator  logicop=OR  UseBitMask=off  NumInputPorts=2  BitMask=double(0)  BitMaskRealWorld=Real World Value
  Bit_XOR : simulink/Logic and Bit Operations/Bitwise Operator  logicop=XOR  UseBitMask=off  NumInputPorts=2  BitMask=double(0)  BitMaskRealWorld=Real World Value
  Bit_XOR_1 : simulink/Logic and Bit Operations/Bitwise Operator  logicop=XOR  UseBitMask=off  NumInputPorts=2  BitMask=double(0)  BitMaskRealWorld=Real World Value
  Bit_XOR_2 : simulink/Logic and Bit Operations/Bitwise Operator  logicop=XOR  UseBitMask=off  NumInputPorts=2  BitMask=double(0)  BitMaskRealWorld=Real World Value
  S : Outport  OutDataTypeStr=fixdt(0, 1, 0)  SampleTime=-1
  C : Outport  Port=2  OutDataTypeStr=fixdt(0, 1, 0)  SampleTime=-1
  wires:
  in1/1 -> Bit_XOR_2/1, Bit_AND/1, Bit_XOR_1/1
  Cin/1 -> Bit_AND_1/1, Bit_XOR/2
  Bit_AND_1/1 -> Bit_OR/2
  Bit_OR/1 -> C/1
  in2/1 -> Bit_XOR_2/2, Bit_AND/2, Bit_XOR_1/2
  Bit_AND/1 -> Bit_OR/1
  Bit_XOR_2/1 -> Bit_AND_1/2
  Bit_XOR/1 -> S/1
  Bit_XOR_1/1 -> Bit_XOR/1

== system wt_multi/wt_multi/ca05/fa ==
  in1 : Inport  OutDataTypeStr=fixdt(0, 1, 0)  SampleTime=-1
  in2 : Inport  Port=2  OutDataTypeStr=fixdt(0, 1, 0)  SampleTime=-1
  Cin : Inport  Port=3  OutDataTypeStr=fixdt(0, 1, 0)  SampleTime=-1
  Bit_AND : simulink/Logic and Bit Operations/Bitwise Operator  logicop=AND  UseBitMask=off  NumInputPorts=2  BitMask=double(0)  BitMaskRealWorld=Real World Value
  Bit_AND_1 : simulink/Logic and Bit Operations/Bitwise Operator  logicop=AND  UseBitMask=off  NumInputPorts=2  BitMask=double(0)  BitMaskRealWorld=Real World Value
  Bit_OR : simulink/Logic and Bit Operations/Bitwise Operator  logicop=OR  UseBitMask=off  NumInputPorts=2  BitMask=double(0)  BitMaskRealWorld=Real World Value
  Bit_XOR : simulink/Logic and Bit Operations/Bitwise Operator  logicop=XOR  UseBitMask=off  NumInputPorts=2  BitMask=double(0)  BitMaskRealWorld=Real World Value
  Bit_XOR_1 : simulink/Logic and Bit Operations/Bitwise Operator  logicop=XOR  UseBitMask=off  NumInputPorts=2  BitMask=double(0)  BitMaskRealWorld=Real World Value
  Bit_XOR_2 : simulink/Logic and Bit Operations/Bitwise Operator  logicop=XOR  UseBitMask=off  NumInputPorts=2  BitMask=double(0)  BitMaskRealWorld=Real World Value
  S : Outport  OutDataTypeStr=fixdt(0, 1, 0)  SampleTime=-1
  C : Outport  Port=2  OutDataTypeStr=fixdt(0, 1, 0)  SampleTime=-1
  wires:
  in1/1 -> Bit_XOR_2/1, Bit_AND/1, Bit_XOR_1/1
  in2/1 -> Bit_XOR_2/2, Bit_AND/2, Bit_XOR_1/2
  Cin/1 -> Bit_AND_1/1, Bit_XOR/2
  Bit_AND_1/1 -> Bit_OR/2
  Bit_OR/1 -> C/1
  Bit_XOR_2/1 -> Bit_AND_1/2
  Bit_XOR/1 -> S/1
  Bit_AND/1 -> Bit_OR/1
  Bit_XOR_1/1 -> Bit_XOR/1

== system wt_multi/wt_multi/ca05/fa1 ==
  in1 : Inport  OutDataTypeStr=fixdt(0, 1, 0)  SampleTime=-1
  in2 : Inport  Port=2  OutDataTypeStr=fixdt(0, 1, 0)  SampleTime=-1
  Cin : Inport  Port=3  OutDataTypeStr=fixdt(0, 1, 0)  SampleTime=-1
  Bit_AND : simulink/Logic and Bit Operations/Bitwise Operator  logicop=AND  UseBitMask=off  NumInputPorts=2  BitMask=double(0)  BitMaskRealWorld=Real World Value
  Bit_AND_1 : simulink/Logic and Bit Operations/Bitwise Operator  logicop=AND  UseBitMask=off  NumInputPorts=2  BitMask=double(0)  BitMaskRealWorld=Real World Value
  Bit_OR : simulink/Logic and Bit Operations/Bitwise Operator  logicop=OR  UseBitMask=off  NumInputPorts=2  BitMask=double(0)  BitMaskRealWorld=Real World Value
  Bit_XOR : simulink/Logic and Bit Operations/Bitwise Operator  logicop=XOR  UseBitMask=off  NumInputPorts=2  BitMask=double(0)  BitMaskRealWorld=Real World Value
  Bit_XOR_1 : simulink/Logic and Bit Operations/Bitwise Operator  logicop=XOR  UseBitMask=off  NumInputPorts=2  BitMask=double(0)  BitMaskRealWorld=Real World Value
  Bit_XOR_2 : simulink/Logic and Bit Operations/Bitwise Operator  logicop=XOR  UseBitMask=off  NumInputPorts=2  BitMask=double(0)  BitMaskRealWorld=Real World Value
  S : Outport  OutDataTypeStr=fixdt(0, 1, 0)  SampleTime=-1
  C : Outport  Port=2  OutDataTypeStr=fixdt(0, 1, 0)  SampleTime=-1
  wires:
  in1/1 -> Bit_XOR_2/1, Bit_AND/1, Bit_XOR_1/1
  in2/1 -> Bit_XOR_2/2, Bit_AND/2, Bit_XOR_1/2
  Cin/1 -> Bit_AND_1/1, Bit_XOR/2
  Bit_AND_1/1 -> Bit_OR/2
  Bit_OR/1 -> C/1
  Bit_AND/1 -> Bit_OR/1
  Bit_XOR_2/1 -> Bit_AND_1/2
  Bit_XOR/1 -> S/1
  Bit_XOR_1/1 -> Bit_XOR/1

== system wt_multi/wt_multi/ca05/fa10 ==
  in1 : Inport  OutDataTypeStr=fixdt(0, 1, 0)  SampleTime=-1
  in2 : Inport  Port=2  OutDataTypeStr=fixdt(0, 1, 0)  SampleTime=-1
  Cin : Inport  Port=3  OutDataTypeStr=fixdt(0, 1, 0)  SampleTime=-1
  Bit_AND : simulink/Logic and Bit Operations/Bitwise Operator  logicop=AND  UseBitMask=off  NumInputPorts=2  BitMask=double(0)  BitMaskRealWorld=Real World Value
  Bit_AND_1 : simulink/Logic and Bit Operations/Bitwise Operator  logicop=AND  UseBitMask=off  NumInputPorts=2  BitMask=double(0)  BitMaskRealWorld=Real World Value
  Bit_OR : simulink/Logic and Bit Operations/Bitwise Operator  logicop=OR  UseBitMask=off  NumInputPorts=2  BitMask=double(0)  BitMaskRealWorld=Real World Value
  Bit_XOR : simulink/Logic and Bit Operations/Bitwise Operator  logicop=XOR  UseBitMask=off  NumInputPorts=2  BitMask=double(0)  BitMaskRealWorld=Real World Value
  Bit_XOR_1 : simulink/Logic and Bit Operations/Bitwise Operator  logicop=XOR  UseBitMask=off  NumInputPorts=2  BitMask=double(0)  BitMaskRealWorld=Real World Value
  Bit_XOR_2 : simulink/Logic and Bit Operations/Bitwise Operator  logicop=XOR  UseBitMask=off  NumInputPorts=2  BitMask=double(0)  BitMaskRealWorld=Real World Value
  S : Outport  OutDataTypeStr=fixdt(0, 1, 0)  SampleTime=-1
  C : Outport  Port=2  OutDataTypeStr=fixdt(0, 1, 0)  SampleTime=-1
  wires:
  Cin/1 -> Bit_AND_1/1, Bit_XOR/2
  in2/1 -> Bit_XOR_2/2, Bit_AND/2, Bit_XOR_1/2
  Bit_AND_1/1 -> Bit_OR/2
  Bit_AND/1 -> Bit_OR/1
  Bit_XOR_2/1 -> Bit_AND_1/2
  Bit_XOR/1 -> S/1
  in1/1 -> Bit_XOR_2/1, Bit_AND/1, Bit_XOR_1/1
  Bit_OR/1 -> C/1
  Bit_XOR_1/1 -> Bit_XOR/1

== system wt_multi/wt_multi/ca05/fa11 ==
  in1 : Inport  OutDataTypeStr=fixdt(0, 1, 0)  SampleTime=-1
  in2 : Inport  Port=2  OutDataTypeStr=fixdt(0, 1, 0)  SampleTime=-1
  Cin : Inport  Port=3  OutDataTypeStr=fixdt(0, 1, 0)  SampleTime=-1
  Bit_AND : simulink/Logic and Bit Operations/Bitwise Operator  logicop=AND  UseBitMask=off  NumInputPorts=2  BitMask=double(0)  BitMaskRealWorld=Real World Value
  Bit_AND_1 : simulink/Logic and Bit Operations/Bitwise Operator  logicop=AND  UseBitMask=off  NumInputPorts=2  BitMask=double(0)  BitMaskRealWorld=Real World Value
  Bit_OR : simulink/Logic and Bit Operations/Bitwise Operator  logicop=OR  UseBitMask=off  NumInputPorts=2  BitMask=double(0)  BitMaskRealWorld=Real World Value
  Bit_XOR : simulink/Logic and Bit Operations/Bitwise Operator  logicop=XOR  UseBitMask=off  NumInputPorts=2  BitMask=double(0)  BitMaskRealWorld=Real World Value
  Bit_XOR_1 : simulink/Logic and Bit Operations/Bitwise Operator  logicop=XOR  UseBitMask=off  NumInputPorts=2  BitMask=double(0)  BitMaskRealWorld=Real World Value
  Bit_XOR_2 : simulink/Logic and Bit Operations/Bitwise Operator  logicop=XOR  UseBitMask=off  NumInputPorts=2  BitMask=double(0)  BitMaskRealWorld=Real World Value
  S : Outport  OutDataTypeStr=fixdt(0, 1, 0)  SampleTime=-1
  C : Outport  Port=2  OutDataTypeStr=fixdt(0, 1, 0)  SampleTime=-1
  wires:
  in1/1 -> Bit_XOR_2/1, Bit_AND/1, Bit_XOR_1/1
  in2/1 -> Bit_XOR_2/2, Bit_AND/2, Bit_XOR_1/2
  Cin/1 -> Bit_AND_1/1, Bit_XOR/2
  Bit_AND_1/1 -> Bit_OR/2
  Bit_OR/1 -> C/1
  Bit_XOR_2/1 -> Bit_AND_1/2
  Bit_AND/1 -> Bit_OR/1
  Bit_XOR/1 -> S/1
  Bit_XOR_1/1 -> Bit_XOR/1

== system wt_multi/wt_multi/ca05/fa12 ==
  in1 : Inport  OutDataTypeStr=fixdt(0, 1, 0)  SampleTime=-1
  in2 : Inport  Port=2  OutDataTypeStr=fixdt(0, 1, 0)  SampleTime=-1
  Cin : Inport  Port=3  OutDataTypeStr=fixdt(0, 1, 0)  SampleTime=-1
  Bit_AND : simulink/Logic and Bit Operations/Bitwise Operator  logicop=AND  UseBitMask=off  NumInputPorts=2  BitMask=double(0)  BitMaskRealWorld=Real World Value
  Bit_AND_1 : simulink/Logic and Bit Operations/Bitwise Operator  logicop=AND  UseBitMask=off  NumInputPorts=2  BitMask=double(0)  BitMaskRealWorld=Real World Value
  Bit_OR : simulink/Logic and Bit Operations/Bitwise Operator  logicop=OR  UseBitMask=off  NumInputPorts=2  BitMask=double(0)  BitMaskRealWorld=Real World Value
  Bit_XOR : simulink/Logic and Bit Operations/Bitwise Operator  logicop=XOR  UseBitMask=off  NumInputPorts=2  BitMask=double(0)  BitMaskRealWorld=Real World Value
  Bit_XOR_1 : simulink/Logic and Bit Operations/Bitwise Operator  logicop=XOR  UseBitMask=off  NumInputPorts=2  BitMask=double(0)  BitMaskRealWorld=Real World Value
  Bit_XOR_2 : simulink/Logic and Bit Operations/Bitwise Operator  logicop=XOR  UseBitMask=off  NumInputPorts=2  BitMask=double(0)  BitMaskRealWorld=Real World Value
  S : Outport  OutDataTypeStr=fixdt(0, 1, 0)  SampleTime=-1
  C : Outport  Port=2  OutDataTypeStr=fixdt(0, 1, 0)  SampleTime=-1
  wires:
  in2/1 -> Bit_XOR_2/2, Bit_AND/2, Bit_XOR_1/2
  Cin/1 -> Bit_AND_1/1, Bit_XOR/2
  in1/1 -> Bit_XOR_2/1, Bit_AND/1, Bit_XOR_1/1
  Bit_AND_1/1 -> Bit_OR/2
  Bit_XOR/1 -> S/1
  Bit_OR/1 -> C/1
  Bit_XOR_2/1 -> Bit_AND_1/2
  Bit_AND/1 -> Bit_OR/1
  Bit_XOR_1/1 -> Bit_XOR/1

== system wt_multi/wt_multi/ca05/fa13 ==
  in1 : Inport  OutDataTypeStr=fixdt(0, 1, 0)  SampleTime=-1
  in2 : Inport  Port=2  OutDataTypeStr=fixdt(0, 1, 0)  SampleTime=-1
  Cin : Inport  Port=3  OutDataTypeStr=fixdt(0, 1, 0)  SampleTime=-1
  Bit_AND : simulink/Logic and Bit Operations/Bitwise Operator  logicop=AND  UseBitMask=off  NumInputPorts=2  BitMask=double(0)  BitMaskRealWorld=Real World Value
  Bit_AND_1 : simulink/Logic and Bit Operations/Bitwise Operator  logicop=AND  UseBitMask=off  NumInputPorts=2  BitMask=double(0)  BitMaskRealWorld=Real World Value
  Bit_OR : simulink/Logic and Bit Operations/Bitwise Operator  logicop=OR  UseBitMask=off  NumInputPorts=2  BitMask=double(0)  BitMaskRealWorld=Real World Value
  Bit_XOR : simulink/Logic and Bit Operations/Bitwise Operator  logicop=XOR  UseBitMask=off  NumInputPorts=2  BitMask=double(0)  BitMaskRealWorld=Real World Value
  Bit_XOR_1 : simulink/Logic and Bit Operations/Bitwise Operator  logicop=XOR  UseBitMask=off  NumInputPorts=2  BitMask=double(0)  BitMaskRealWorld=Real World Value
  Bit_XOR_2 : simulink/Logic and Bit Operations/Bitwise Operator  logicop=XOR  UseBitMask=off  NumInputPorts=2  BitMask=double(0)  BitMaskRealWorld=Real World Value
  S : Outport  OutDataTypeStr=fixdt(0, 1, 0)  SampleTime=-1
  C : Outport  Port=2  OutDataTypeStr=fixdt(0, 1, 0)  SampleTime=-1
  wires:
  in1/1 -> Bit_XOR_2/1, Bit_AND/1, Bit_XOR_1/1
  in2/1 -> Bit_XOR_2/2, Bit_AND/2, Bit_XOR_1/2
  Cin/1 -> Bit_AND_1/1, Bit_XOR/2
  Bit_AND_1/1 -> Bit_OR/2
  Bit_OR/1 -> C/1
  Bit_XOR_1/1 -> Bit_XOR/1
  Bit_XOR_2/1 -> Bit_AND_1/2
  Bit_AND/1 -> Bit_OR/1
  Bit_XOR/1 -> S/1

== system wt_multi/wt_multi/ca05/fa14 ==
  in1 : Inport  OutDataTypeStr=fixdt(0, 1, 0)  SampleTime=-1
  in2 : Inport  Port=2  OutDataTypeStr=fixdt(0, 1, 0)  SampleTime=-1
  Cin : Inport  Port=3  OutDataTypeStr=fixdt(0, 1, 0)  SampleTime=-1
  Bit_AND : simulink/Logic and Bit Operations/Bitwise Operator  logicop=AND  UseBitMask=off  NumInputPorts=2  BitMask=double(0)  BitMaskRealWorld=Real World Value
  Bit_AND_1 : simulink/Logic and Bit Operations/Bitwise Operator  logicop=AND  UseBitMask=off  NumInputPorts=2  BitMask=double(0)  BitMaskRealWorld=Real World Value
  Bit_OR : simulink/Logic and Bit Operations/Bitwise Operator  logicop=OR  UseBitMask=off  NumInputPorts=2  BitMask=double(0)  BitMaskRealWorld=Real World Value
  Bit_XOR : simulink/Logic and Bit Operations/Bitwise Operator  logicop=XOR  UseBitMask=off  NumInputPorts=2  BitMask=double(0)  BitMaskRealWorld=Real World Value
  Bit_XOR_1 : simulink/Logic and Bit Operations/Bitwise Operator  logicop=XOR  UseBitMask=off  NumInputPorts=2  BitMask=double(0)  BitMaskRealWorld=Real World Value
  Bit_XOR_2 : simulink/Logic and Bit Operations/Bitwise Operator  logicop=XOR  UseBitMask=off  NumInputPorts=2  BitMask=double(0)  BitMaskRealWorld=Real World Value
  S : Outport  OutDataTypeStr=fixdt(0, 1, 0)  SampleTime=-1
  C : Outport  Port=2  OutDataTypeStr=fixdt(0, 1, 0)  SampleTime=-1
  wires:
  in1/1 -> Bit_XOR_2/1, Bit_AND/1, Bit_XOR_1/1
  in2/1 -> Bit_XOR_2/2, Bit_AND/2, Bit_XOR_1/2
  Cin/1 -> Bit_AND_1/1, Bit_XOR/2
  Bit_AND_1/1 -> Bit_OR/2
  Bit_XOR_2/1 -> Bit_AND_1/2
  Bit_OR/1 -> C/1
  Bit_XOR_1/1 -> Bit_XOR/1
  Bit_AND/1 -> Bit_OR/1
  Bit_XOR/1 -> S/1

== system wt_multi/wt_multi/ca05/fa15 ==
  in1 : Inport  OutDataTypeStr=fixdt(0, 1, 0)  SampleTime=-1
  in2 : Inport  Port=2  OutDataTypeStr=fixdt(0, 1, 0)  SampleTime=-1
  Cin : Inport  Port=3  OutDataTypeStr=fixdt(0, 1, 0)  SampleTime=-1
  Bit_AND : simulink/Logic and Bit Operations/Bitwise Operator  logicop=AND  UseBitMask=off  NumInputPorts=2  BitMask=double(0)  BitMaskRealWorld=Real World Value
  Bit_AND_1 : simulink/Logic and Bit Operations/Bitwise Operator  logicop=AND  UseBitMask=off  NumInputPorts=2  BitMask=double(0)  BitMaskRealWorld=Real World Value
  Bit_OR : simulink/Logic and Bit Operations/Bitwise Operator  logicop=OR  UseBitMask=off  NumInputPorts=2  BitMask=double(0)  BitMaskRealWorld=Real World Value
  Bit_XOR : simulink/Logic and Bit Operations/Bitwise Operator  logicop=XOR  UseBitMask=off  NumInputPorts=2  BitMask=double(0)  BitMaskRealWorld=Real World Value
  Bit_XOR_1 : simulink/Logic and Bit Operations/Bitwise Operator  logicop=XOR  UseBitMask=off  NumInputPorts=2  BitMask=double(0)  BitMaskRealWorld=Real World Value
  Bit_XOR_2 : simulink/Logic and Bit Operations/Bitwise Operator  logicop=XOR  UseBitMask=off  NumInputPorts=2  BitMask=double(0)  BitMaskRealWorld=Real World Value
  S : Outport  OutDataTypeStr=fixdt(0, 1, 0)  SampleTime=-1
  C : Outport  Port=2  OutDataTypeStr=fixdt(0, 1, 0)  SampleTime=-1
  wires:
  in1/1 -> Bit_XOR_2/1, Bit_AND/1, Bit_XOR_1/1
  in2/1 -> Bit_XOR_2/2, Bit_AND/2, Bit_XOR_1/2
  Cin/1 -> Bit_AND_1/1, Bit_XOR/2
  Bit_OR/1 -> C/1
  Bit_AND_1/1 -> Bit_OR/2
  Bit_XOR/1 -> S/1
  Bit_XOR_2/1 -> Bit_AND_1/2
  Bit_XOR_1/1 -> Bit_XOR/1
  Bit_AND/1 -> Bit_OR/1

== system wt_multi/wt_multi/ca05/fa16 ==
  in1 : Inport  OutDataTypeStr=fixdt(0, 1, 0)  SampleTime=-1
  in2 : Inport  Port=2  OutDataTypeStr=fixdt(0, 1, 0)  SampleTime=-1
  Cin : Inport  Port=3  OutDataTypeStr=fixdt(0, 1, 0)  SampleTime=-1
  Bit_AND : simulink/Logic and Bit Operations/Bitwise Operator  logicop=AND  UseBitMask=off  NumInputPorts=2  BitMask=double(0)  BitMaskRealWorld=Real World Value
  Bit_AND_1 : simulink/Logic and Bit Operations/Bitwise Operator  logicop=AND  UseBitMask=off  NumInputPorts=2  BitMask=double(0)  BitMaskRealWorld=Real World Value
  Bit_OR : simulink/Logic and Bit Operations/Bitwise Operator  logicop=OR  UseBitMask=off  NumInputPorts=2  BitMask=double(0)  BitMaskRealWorld=Real World Value
  Bit_XOR : simulink/Logic and Bit Operations/Bitwise Operator  logicop=XOR  UseBitMask=off  NumInputPorts=2  BitMask=double(0)  BitMaskRealWorld=Real World Value
  Bit_XOR_1 : simulink/Logic and Bit Operations/Bitwise Operator  logicop=XOR  UseBitMask=off  NumInputPorts=2  BitMask=double(0)  BitMaskRealWorld=Real World Value
  Bit_XOR_2 : simulink/Logic and Bit Operations/Bitwise Operator  logicop=XOR  UseBitMask=off  NumInputPorts=2  BitMask=double(0)  BitMaskRealWorld=Real World Value
  S : Outport  OutDataTypeStr=fixdt(0, 1, 0)  SampleTime=-1
  C : Outport  Port=2  OutDataTypeStr=fixdt(0, 1, 0)  SampleTime=-1
  wires:
  in2/1 -> Bit_XOR_2/2, Bit_AND/2, Bit_XOR_1/2
  Bit_AND_1/1 -> Bit_OR/2
  Bit_OR/1 -> C/1
  Cin/1 -> Bit_AND_1/1, Bit_XOR/2
  Bit_AND/1 -> Bit_OR/1
  Bit_XOR/1 -> S/1
  Bit_XOR_2/1 -> Bit_AND_1/2
  in1/1 -> Bit_XOR_2/1, Bit_AND/1, Bit_XOR_1/1
  Bit_XOR_1/1 -> Bit_XOR/1
